simulink subsystem "Sensors"  (R2020a)
settings: Solver=VariableStepAuto  StartTime=0.0  StopTime=10.0  RelTol=1e-3
settings Model: Creator=decla  LastModifiedBy=decla

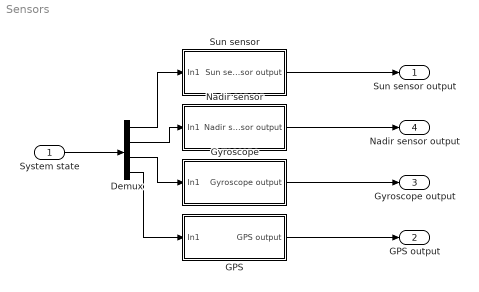
== system Sensors ==
  System state : Inport
  Demux : Demux
  GPS : Subsystem
  Gyroscope : Subsystem
  Nadir sensor : Subsystem
  Sun sensor : Subsystem
  Sun sensor output : Outport
  GPS output : Outport  Port=2
  Gyroscope output : Outport  Port=3
  Nadir sensor output : Outport  Port=4
  wires:
  System state/1 -> Demux/1
  Demux/1 -> Sun sensor/1(In1)
  Demux/2 -> Nadir sensor/1(In1)
  Demux/3 -> Gyroscope/1(In1)
  Demux/4 -> GPS/1(In1)
  Sun sensor/1(Sun sensor output) -> Sun sensor output/1
  Nadir sensor/1(Nadir sensor output) -> Nadir sensor output/1
  Gyroscope/1(Gyroscope output) -> Gyroscope output/1
  GPS/1(GPS output) -> GPS output/1

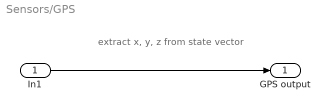
== system Sensors/GPS ==
  note: extract x, y, z from state vector
  In1 : Inport
  GPS output : Outport
  wires:
  In1/1 -> GPS output/1

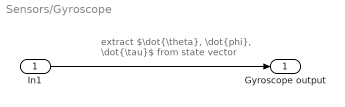
== system Sensors/Gyroscope ==
  note: extract $\dot{\theta}, \dot{phi}, \dot{\tau}$ from state vector
  In1 : Inport
  Gyroscope output : Outport
  wires:
  In1/1 -> Gyroscope output/1

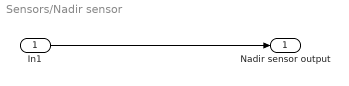
== system Sensors/Nadir sensor ==
  In1 : Inport
  Nadir sensor output : Outport
  wires:
  In1/1 -> Nadir sensor output/1

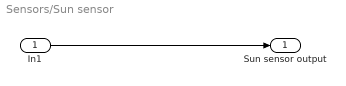
== system Sensors/Sun sensor ==
  In1 : Inport
  Sun sensor output : Outport
  wires:
  In1/1 -> Sun sensor output/1
